simulink model "Super11_tmp"  (Simulink 8.3)
settings: Solver=FixedStepDiscrete  StartTime=0.0  StopTime=10.0  RelTol=1e-3
settings Model: Creator=scaife  LastModifiedBy=bourbouh  CovSFcnEnable=on  ExtModeAutoUpdateStatusClock=off
settings DataIOCC: SignalLoggingName=sigsOut
settings DebuggingCC: SaveWithParameterizedLinksMsg=none  SignalResolutionControl=TryResolveAllWithWarning  SolverPrmCheckMsg=none  MultiTaskDSMMsg=warning  MultiTaskCondExecSysMsg=none  FrameProcessingCompatibilityMsg=error  StateNameClashWarn=none
settings HardwareCC: TargetUnknown=on
settings SFSimCC: SimParseCustomCode=off

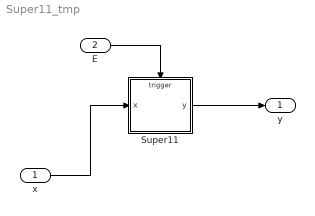
== system Super11_tmp ==
  x : Inport
  E : Inport  Port=2
  Super11 : Stateflow chart  TreatAsAtomicUnit=on
      settings: PermitHierarchicalResolution=ParametersOnly
  y : Outport
  wires:
  x/1 -> Super11/1(x)
  Super11/1(y) -> y/1
  E/1 -> Super11/Trigger

== stateflow chart Super11 ==
  state A
    du : y++;
  state B
    du : y++;
    state B1
      du : y++;
    state B2
      du : y++;
      state B2a
        du : y++;
      (default) -> B2a
      B2a -> (junction 11) : E
    (default) -> B1
    B1 -> B2 : E
    (junction 11) -> B1 [order 2] : [x<>0]
  (junction 17) -> B [order 1] : [x==0]
  A -> (junction 17) : E
  (junction 17) -> B2a [order 2] : [x<>0]
  (junction 11) -> A [order 1] : [x==0]
  (default) -> A
  data: x input int8; y output uint32
  events: E input EITHER_EDGE_EVENT
